simulink model "intrinsicStiffnessLPVModel"  (Simulink 8.2)
settings: Solver=ode3  StartTime=0.0  StopTime=59.999  FixedStep=0.001  RelTol=1e-3
values from neighbouring files (symbols this model uses):
  h = sign(omega_hat(1,i))    [pcas_short_segment_exp_new_intrinsic_irf1.m]    (also in simulateIntrinsic.m = irfModel.dataSet; simulate_LPV_ParallelCascade.m = irfModel.dataSet)
settings Model: Creator=Kian  LastModifiedBy=Kian
settings DataIOCC: SignalLoggingSaveFormat=Dataset
settings OptimizationCC: ExpressionDepthLimit=128
settings DebuggingCC: FcnCallInpInsideContextMsg=EnableAllAsError  StateNameClashWarn=none
settings GRTTargetCC: CombineOutputUpdateFcns=on  GRTInterface=off

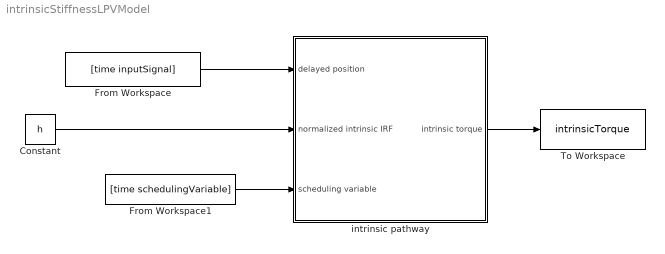
== system intrinsicStiffnessLPVModel ==
  Constant : Constant  Value=h
  From Workspace : FromWorkspace  VariableName=[time inputSignal]  SampleTime=.001
  From Workspace1 : FromWorkspace  VariableName=[time schedulingVariable]  SampleTime=0.001
  To Workspace : ToWorkspace  VariableName=intrinsicTorque  SampleTime=-1  SaveFormat=Timeseries
  "intrinsic pathway " : Subsystem
  wires:
  From Workspace/1 -> "intrinsic pathway "/1(delayed position)
  Constant/1 -> "intrinsic pathway "/2(normalized intrinsic IRF)
  From Workspace1/1 -> "intrinsic pathway "/3(scheduling variable)
  "intrinsic pathway "/1(intrinsic torque) -> To Workspace/1

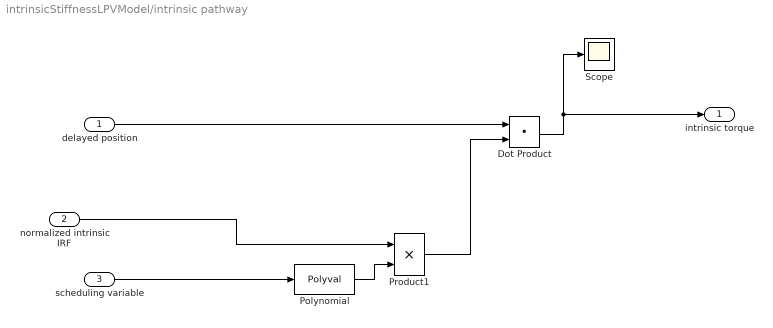
== system intrinsicStiffnessLPVModel/intrinsic pathway  ==
  delayed position : Inport
  normalized intrinsic IRF : Inport  Port=2
  scheduling variable : Inport  Port=3
  Dot Product : DotProduct  InputSameDT=on  OutDataTypeStr=Inherit: Inherit via internal rule
  Polynomial : Polyval  Coefs=[ +2.081618890e-019, -1.441693666e-014, +4.719686976e-010, -8.536869453e-006, +1.621573104e-001, -8.087801117e+001 ]
  Product1 : Product
  Scope : Scope
  intrinsic torque : Outport
  wires:
  delayed position/1 -> Dot Product/1
  scheduling variable/1 -> Polynomial/1
  Dot Product/1 -> intrinsic torque/1, Scope/1
  Product1/1 -> Dot Product/2
  normalized intrinsic IRF/1 -> Product1/1
  Polynomial/1 -> Product1/2
